simulink model "sim_mobile_robot_trajectory_control_pid"  (R2020b)
settings: Solver=ode1  StartTime=0.0  StopTime=100  FixedStep=0.01  RelTol=1e-3
undefined symbols (not defined in the file): a, b, Kd, Ki, Kp
libraries: simulink x2, dspsigops x1
settings Model: Creator=ONLY-GOD  LastModifiedBy=ONLY-GOD

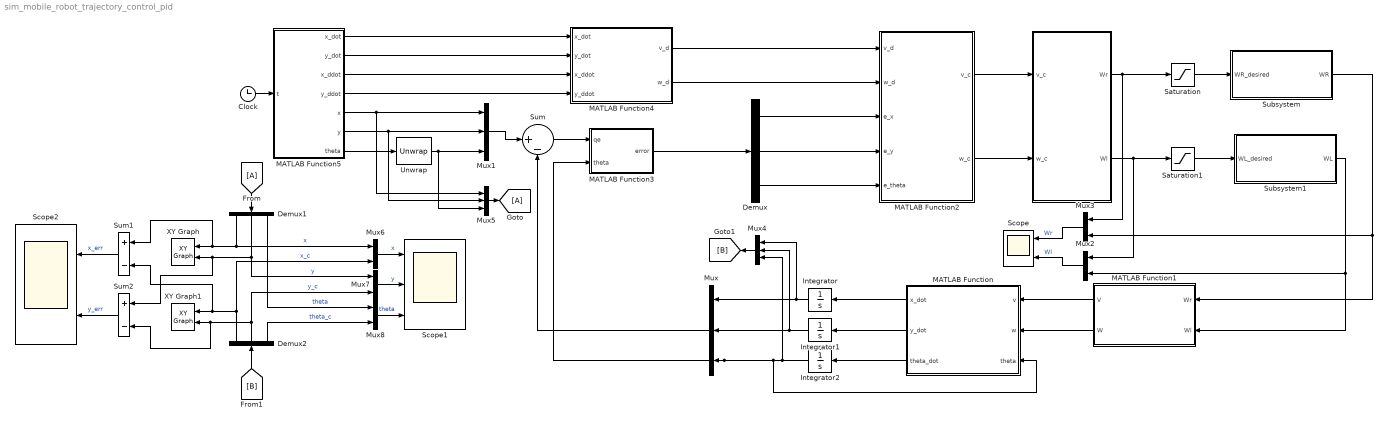
== system sim_mobile_robot_trajectory_control_pid ==
  " " : MATLAB Function  TreatAsAtomicUnit=on
  Clock : Clock
  Demux : Demux  Outputs=3
  Demux1 : Demux  Outputs=3
  Demux2 : Demux  Outputs=3
  Integrator : Integrator
  Integrator1 : Integrator
  Integrator2 : Integrator
  MATLAB Function : MATLAB Function  TreatAsAtomicUnit=on
  MATLAB Function1 : MATLAB Function  TreatAsAtomicUnit=on
  MATLAB Function2 : MATLAB Function  TreatAsAtomicUnit=on
  MATLAB Function3 : MATLAB Function  TreatAsAtomicUnit=on
  MATLAB Function4 : MATLAB Function  TreatAsAtomicUnit=on
  MATLAB Function5 : MATLAB Function  TreatAsAtomicUnit=on
  Mux{,1,4..5} (4 alike) : Mux  Inputs=3
  Mux{2..3,6..8} (5 alike) : Mux  Inputs=2
  Saturation : Saturate  UpperLimit=14  LowerLimit=-14
  Saturation1 : Saturate  UpperLimit=14  LowerLimit=-14
  Scope : Scope  NumInputPorts=2
  Scope1 : Scope  NumInputPorts=3
  Scope2 : Scope  NumInputPorts=2
  Subsystem : Subsystem
  Subsystem1 : Subsystem
  Sum : Sum  Inputs=|+-
  Sum1 : Sum  Inputs=+-
  Sum2 : Sum  Inputs=+-
  Unwrap : dspsigops/Unwrap  tol=pi  InputProcessing=Columns as channels (frame based)  running=off
  XY Graph : simulink/Sinks/XY Graph  xmin=-6  xmax=6  ymin=-6  ymax=6  st=-1
  XY Graph1 : simulink/Sinks/XY Graph  xmin=-6  xmax=6  ymin=-6  ymax=6  st=-1
  wires:
  Demux/1 -> MATLAB Function2/3(e_x)
  Demux/2 -> MATLAB Function2/4(e_y)
  Demux/3 -> MATLAB Function2/5(e_theta)
  Sum/1 -> MATLAB Function3/1(qe)
  MATLAB Function3/1(error) -> Demux/1
  MATLAB Function4/1(v_d) -> MATLAB Function2/1(v_d)
  MATLAB Function4/2(w_d) -> MATLAB Function2/2(w_d)
  MATLAB Function2/1(v_c) -> " "/1(v_c)
  MATLAB Function2/2(w_c) -> " "/2(w_c)
  " "/1(Wr) -> Saturation/1, Mux3/1
  " "/2(Wl) -> Saturation1/1, Mux2/1
  Subsystem/1(WR) -> Mux3/2, MATLAB Function1/1(Wr)
  Subsystem1/1(WL) -> Mux2/2, MATLAB Function1/2(Wl)
  MATLAB Function1/1(V) -> MATLAB Function/1(v)
  MATLAB Function1/2(W) -> MATLAB Function/2(w)
  MATLAB Function/3(theta_dot) -> Integrator2/1
  MATLAB Function/1(x_dot) -> Integrator/1
  MATLAB Function/2(y_dot) -> Integrator1/1
  Integrator2/1 -> Mux4/3, MATLAB Function3/2(theta), Mux/3, MATLAB Function/3(theta)
  Integrator/1 -> Mux4/1, Mux/1
  Integrator1/1 -> Mux4/2, Mux/2
  Mux/1 -> Sum/2
  MATLAB Function5/1(x_dot) -> MATLAB Function4/1(x_dot)
  MATLAB Function5/2(y_dot) -> MATLAB Function4/2(y_dot)
  MATLAB Function5/3(x_ddot) -> MATLAB Function4/3(x_ddot)
  MATLAB Function5/4(y_ddot) -> MATLAB Function4/4(y_ddot)
  Clock/1 -> MATLAB Function5/1(t)
  MATLAB Function5/5(x) -> Mux1/1, Mux5/1
  MATLAB Function5/6(y) -> Mux1/2, Mux5/2
  MATLAB Function5/7(theta) -> Unwrap/1
  Mux1/1 -> Sum/1
  Mux3/1 -> Scope/1  "Wr"
  Mux2/1 -> Scope/2  "Wl"
  Mux5/1 -> [A]
  Mux4/1 -> [B]
  [A] -> Demux1/1
  [B] -> Demux2/1
  Demux1/1 -> Sum1/1, XY Graph/1, Mux6/1  "x"
  Demux2/1 -> XY Graph1/1, Sum1/2, Mux6/2  "x_c"
  Demux1/2 -> Sum2/1, XY Graph/2, Mux7/1  "y"
  Demux2/2 -> Sum2/2, XY Graph1/2, Mux7/2  "y_c"
  Demux2/3 -> Mux8/2  "theta_c"
  Mux6/1 -> Scope1/1  "x"
  Mux7/1 -> Scope1/2  "y"
  Mux8/1 -> Scope1/3  "theta"
  Demux1/3 -> Mux8/1  "theta"
  Sum1/1 -> Scope2/1  "x_err"
  Sum2/1 -> Scope2/2  "y_err"
  Unwrap/1 -> Mux1/3, Mux5/3
  Saturation/1 -> Subsystem/1(WR_desired)
  Saturation1/1 -> Subsystem1/1(WL_desired)

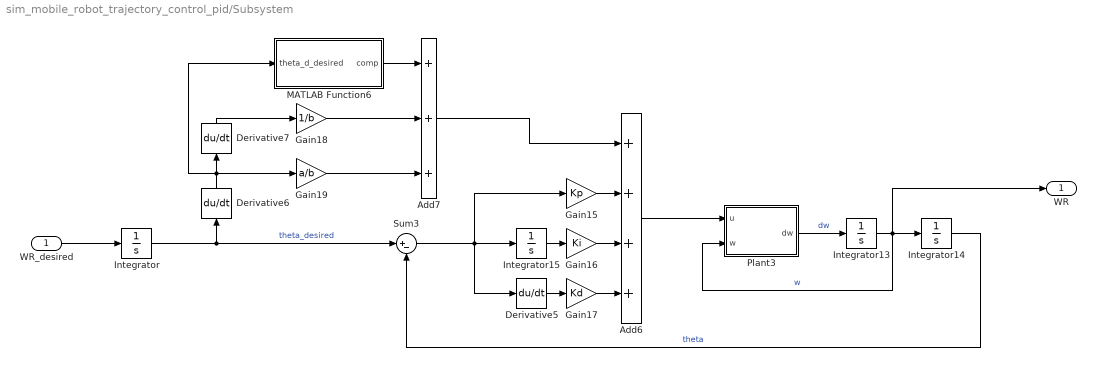
== system sim_mobile_robot_trajectory_control_pid/Subsystem ==
  WR_desired : Inport
  Add6 : Sum  Inputs=++++
  Add7 : Sum  Inputs=+++
  Derivative5 : Derivative
  Derivative6 : Derivative
  Derivative7 : Derivative
  Gain15 : Gain  Gain=Kp
  Gain16 : Gain  Gain=Ki
  Gain17 : Gain  Gain=Kd
  Gain18 : Gain  Gain=1/b
  Gain19 : Gain  Gain=a/b
  Integrator{,13..15} (4 alike) : Integrator
  MATLAB Function6 : MATLAB Function  TreatAsAtomicUnit=on
  Plant3 : MATLAB Function  TreatAsAtomicUnit=on
  Sum3 : Sum  Inputs=|+-
  WR : Outport
  wires:
  Sum3/1 -> Gain15/1, Integrator15/1, Derivative5/1
  Derivative7/1 -> Gain18/1
  Add7/1 -> Add6/1
  Gain17/1 -> Add6/4
  Add6/1 -> Plant3/1(u)
  MATLAB Function6/1(comp) -> Add7/1
  Gain15/1 -> Add6/2
  Integrator13/1 -> WR/1, Integrator14/1, Plant3/2(w)  "w"
  Integrator14/1 -> Sum3/2  "theta"
  Derivative5/1 -> Gain17/1
  Gain18/1 -> Add7/2
  Gain19/1 -> Add7/3
  Integrator15/1 -> Gain16/1
  Gain16/1 -> Add6/3
  Derivative6/1 -> Gain19/1, MATLAB Function6/1(theta_d_desired), Derivative7/1
  Plant3/1(dw) -> Integrator13/1  "dw"
  WR_desired/1 -> Integrator/1
  Integrator/1 -> Sum3/1, Derivative6/1  "theta_desired"

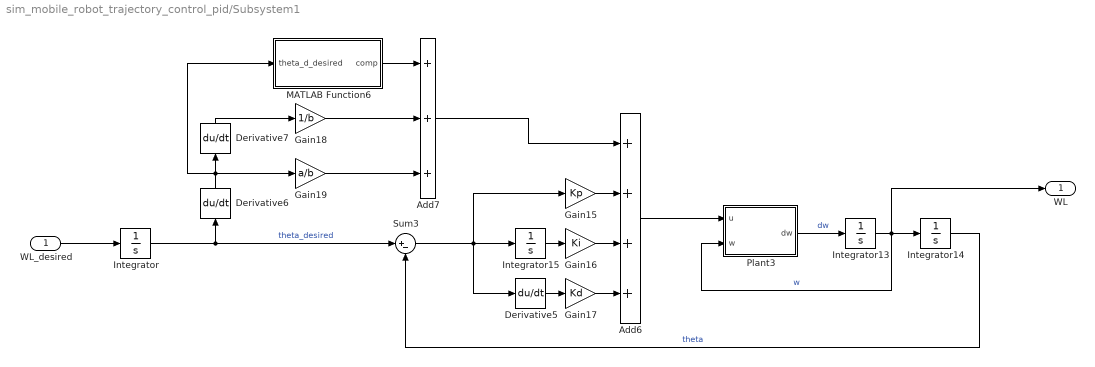
== system sim_mobile_robot_trajectory_control_pid/Subsystem1 ==
  WL_desired : Inport
  Add6 : Sum  Inputs=++++
  Add7 : Sum  Inputs=+++
  Derivative5 : Derivative
  Derivative6 : Derivative
  Derivative7 : Derivative
  Gain15 : Gain  Gain=Kp
  Gain16 : Gain  Gain=Ki
  Gain17 : Gain  Gain=Kd
  Gain18 : Gain  Gain=1/b
  Gain19 : Gain  Gain=a/b
  Integrator{,13..15} (4 alike) : Integrator
  MATLAB Function6 : MATLAB Function  TreatAsAtomicUnit=on
  Plant3 : MATLAB Function  TreatAsAtomicUnit=on
  Sum3 : Sum  Inputs=|+-
  WL : Outport
  wires:
  Integrator/1 -> Derivative6/1, Sum3/1  "theta_desired"
  WL_desired/1 -> Integrator/1
  Plant3/1(dw) -> Integrator13/1  "dw"
  Derivative6/1 -> Derivative7/1, MATLAB Function6/1(theta_d_desired), Gain19/1
  Gain16/1 -> Add6/3
  Integrator15/1 -> Gain16/1
  Gain19/1 -> Add7/3
  Gain18/1 -> Add7/2
  Derivative5/1 -> Gain17/1
  Integrator14/1 -> Sum3/2  "theta"
  Integrator13/1 -> Plant3/2(w), Integrator14/1, WL/1  "w"
  Gain15/1 -> Add6/2
  MATLAB Function6/1(comp) -> Add7/1
  Add6/1 -> Plant3/1(u)
  Gain17/1 -> Add6/4
  Add7/1 -> Add6/1
  Derivative7/1 -> Gain18/1
  Sum3/1 -> Derivative5/1, Integrator15/1, Gain15/1

== matlab function sim_mobile_robot_trajectory_control_pid/  ==
  data: v_c input; Wr output; w_c input; Wl output
function [Wr, Wl] = M_inv(v_c, w_c)
r = 0.07;      %wheel radius
b = 0.22;      %length from wheel to wheel

Wr = ((2*v_c)+(w_c*b))/(2*r);
Wl = ((2*v_c)-(w_c*b))/(2*r);

== matlab function sim_mobile_robot_trajectory_control_pid/Subsystem/Plant3 ==
  settings: updateMethod=DISCRETE
  data: u input; dw output; w input
function dw = dcmotor(u,w)

a = 27.65; b = 17.35; c = 5.63;
dw = -a*w+b*u-c*sign(w) + 1e-4*randn;

== matlab function sim_mobile_robot_trajectory_control_pid/MATLAB Function ==
  data: v input; x_dot output; w input; y_dot output; theta_dot output; theta input
function [x_dot,y_dot,theta_dot]= kinematic(v,w,theta)
x_dot = v*cos(theta);
y_dot = v*sin(theta);
theta_dot = w;

== matlab function sim_mobile_robot_trajectory_control_pid/MATLAB Function2 ==
  data: v_d input; v_c output; w_d input; e_x input; e_y input; e_theta input; w_c output
function [v_c,w_c] =  bckstep(v_d, w_d, e_x, e_y, e_theta)            

% control gain
k1 = 0.1;
k2 = 2 ;
k3 = 1 ;

v_c = k1*e_x + v_d*cos(e_theta);
w_c = w_d + k2*v_d*e_y + k3*v_d*sin(e_theta);

== matlab function sim_mobile_robot_trajectory_control_pid/MATLAB Function3 ==
  data: qe input; error output; theta input
function error = rotation(qe,theta)

T = [cos(theta) , sin(theta) , 0 ;
    -sin(theta) , cos(theta) , 0 ;
         0      ,     0      , 1 ];
     
error = T*qe;

== matlab function sim_mobile_robot_trajectory_control_pid/MATLAB Function4 ==
  data: x_dot input; v_d output; w_d output; y_dot input; x_ddot input; y_ddot input
function [v_d,w_d] = fcn(x_dot,y_dot,x_ddot,y_ddot)

v_d = sqrt(x_dot^2 + y_dot^2);
w_d = ((x_dot*y_ddot)-(y_dot*x_ddot))/((x_dot^2 + y_dot^2));

== matlab function sim_mobile_robot_trajectory_control_pid/Subsystem/MATLAB Function6 ==
  settings: updateMethod=DISCRETE
  data: theta_d_desired input; comp output
function comp = fcn(theta_d_desired)

b = 17.35; c = 5.63; %+ 0.3*rand;
comp = c/b*sign(theta_d_desired);

== matlab function sim_mobile_robot_trajectory_control_pid/Subsystem1/MATLAB Function6 ==
  settings: updateMethod=DISCRETE
  data: theta_d_desired input; comp output
function comp = fcn(theta_d_desired)

b = 17.35; c = 5.63; %+ 0.3*rand;
comp = c/b*sign(theta_d_desired);

== matlab function sim_mobile_robot_trajectory_control_pid/Subsystem1/Plant3 ==
  settings: updateMethod=DISCRETE
  data: u input; dw output; w input
function dw = dcmotor(u,w)

a = 27.65; b = 17.35; c = 5.63;
dw = -a*w+b*u-c*sign(w) + 1e-4*randn;

== matlab function sim_mobile_robot_trajectory_control_pid/MATLAB Function1 ==
  data: Wr input; V output; Wl input; W output
function [V,W]= fcn(Wr,Wl)
r = 0.07;      %wheel radius
b = 0.22;      %length from wheel to wheel

V = r*(Wr/2) + r*(Wl/2);
W = r*(Wr/b) - r*(Wl/b);

== matlab function sim_mobile_robot_trajectory_control_pid/MATLAB Function5 ==
  data: x_dot output; y_dot output; x_ddot output; y_ddot output; x output; t input; y output; theta output
function [x_dot,y_dot,x_ddot,y_ddot,x,y,theta] = ref(t)

f = 2*pi*0.01;
r = 4;

x = r*cos(f*t);
y = r*sin(f*t);

x_dot = -r*f*sin(f*t);
y_dot = r*f*cos(f*t);

theta = atan2(y_dot,x_dot);

x_ddot = -r*f^2*cos(f*t);
y_ddot = -r*f^2*sin(f*t);
